simulink model "galamsey_simulation"  (R2025b)
settings: Solver=VariableStepAuto  StartTime=0.0  StopTime=10.0  RelTol=1e-3
libraries: audiosources x1
settings Model: Creator=Jakabs  LastModifiedBy=Jakabs

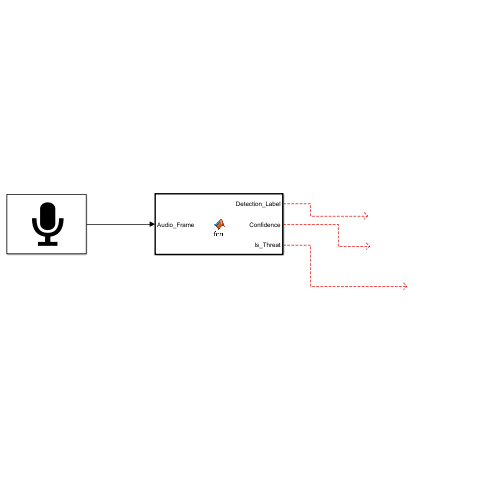
[thumbnail: Simulink's stored preview of the top-level diagram]
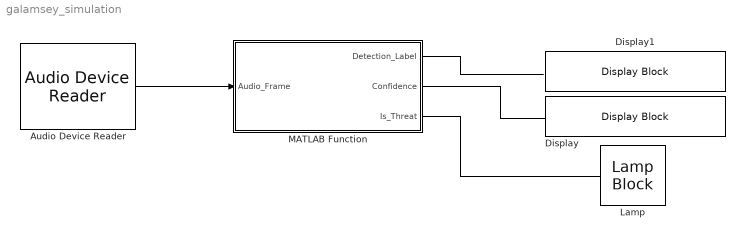
== system galamsey_simulation ==
  Audio Device Reader : audiosources/Audio Device Reader  Driver=DirectSound  Device=Default  SampleRate=22050  NumChannels=1  SamplesPerFrame=33075  BitDepth=16-bit integer  NumBuffers=10  DefaultInputChannelMapping=on  InputChannelMapping=1:2  OutputNumOverrunSamples=off  OutputDataType=double  DriverIdx=1  DeviceWarnFlag=''
  Display : DisplayBlock  LabelPosition=Hide  Transparency=1  GridColor=[0.502, 0.502, 0.502]
  Display1 : DisplayBlock  LabelPosition=Hide  Transparency=1  GridColor=[0.502, 0.502, 0.502]
  Lamp : LampBlock  LabelPosition=Hide  DefaultColor=[192.0, 192.0, 192.0]
  MATLAB Function : MATLAB Function  TreatAsAtomicUnit=on
  wires:
  Audio Device Reader/1 -> MATLAB Function/1(Audio_Frame)
  MATLAB Function/1(Detection_Label) -> ?
  MATLAB Function/2(Confidence) -> ?
  MATLAB Function/3(Is_Threat) -> ?

== matlab function galamsey_simulation/MATLAB Function ==
  data: Audio_Frame input; Detection_Label output; Confidence output; Is_Threat output
function [Detection_Label, Confidence, Is_Threat] = fcn(Audio_Frame)
    % GALAMSEY DETECTOR - STRING OUTPUT VERSION
    
    % 1. Declare the helper function as extrinsic
    coder.extrinsic('run_galamsey_inference');

    % 2. Initialize Outputs
    % We define 'Detection_Label' as a string variable
    Detection_Label = "Initializing..."; 
    Confidence = 0.0;
    Is_Threat = 0;

    % 3. Call the Heavy Logic
    % We use temporary variables for the raw numeric results
    raw_id = 0;
    raw_conf = 0.0;
    raw_threat = 0;
    
    [raw_id, raw_conf, raw_threat] = run_galamsey_inference(Audio_Frame);

    % 4. Convert Numbers to Text
    % Map the ID (1,2,3) to human-readable names
    if raw_id == 2
        Detection_Label = "CHAINSAW";
    elseif raw_id == 3
        Detection_Label = "ENGINE";
    else
        Detection_Label = "Background";
    end

    % 5. Pass through the other data
    Confidence = raw_conf;
    Is_Threat = raw_threat;
end
